simulink model "control_clean"  (R2023a)
settings: Solver=ode1be  StartTime=0.0  StopTime=tf  FixedStep=ts  RelTol=1e-3
values from neighbouring files (symbols this model uses):
  b = 0.41    [parameters.m]
  iz = 4.1    [parameters.m]
  lambda = [lambda_x; lambda_y]    [main.m]
  m = 30    [parameters.m]
  n = 501    [main.m]
  n_r_dot = -2.79    [parameters.m]
  n_v_dot = -16.41    [parameters.m]
  nrr = -3.49    [parameters.m]
  nrv = -8.8    [parameters.m]
  nvr = -8.8    [parameters.m]
  nvv = -5.49    [parameters.m]
  x = x_or    [main.m]
  x_u_dot = -2.25    [parameters.m]
  y = y_or    [main.m]
  y_r_dot = -1.31    [parameters.m]
  y_v_dot = -23.23    [parameters.m]
  yrr = -8.8    [parameters.m]
  yrv = -5.49    [parameters.m]
  yvr = -5.49    [parameters.m]
  yvv = -99.99    [parameters.m]
undefined symbols (not defined in the file or in its folder): l, m_inv
libraries: robotcorelib x1
settings Model: Creator=max  LastModifiedBy=maxpr

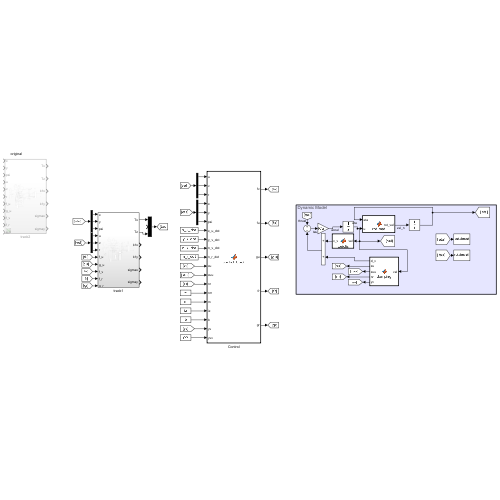
[thumbnail: Simulink's stored preview of the top-level diagram]
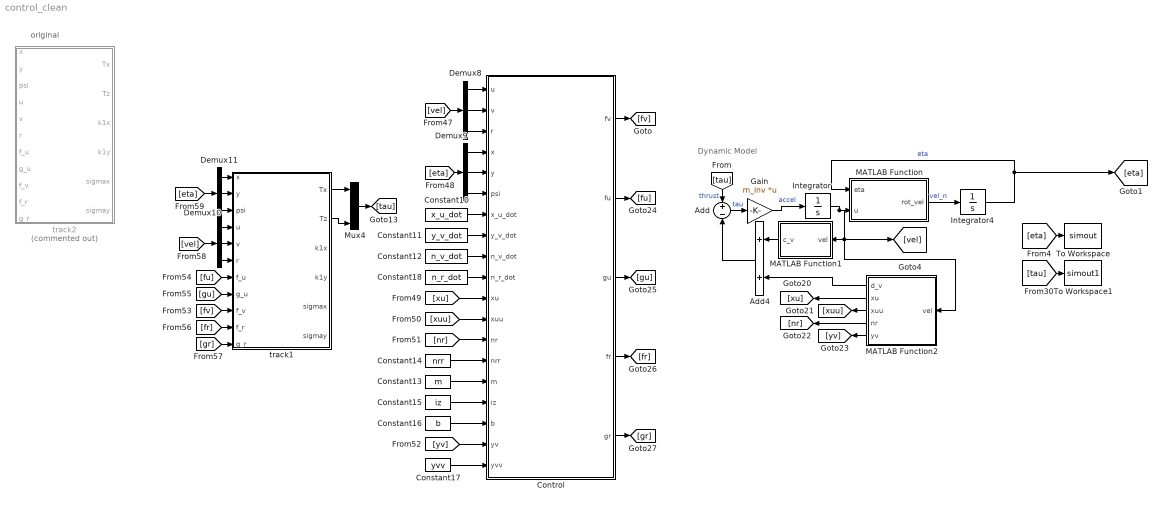
== system control_clean ==
  note: original
  note: Dynamic Model
  Add : Sum  Inputs=+|-
  Add4 : Sum
  Constant10 : Constant  Value=x_u_dot
  Constant11 : Constant  Value=y_v_dot
  Constant12 : Constant  Value=n_v_dot
  Constant13 : Constant  Value=m
  Constant14 : Constant  Value=nrr
  Constant15 : Constant  Value=iz
  Constant16 : Constant  Value=b
  Constant17 : Constant  Value=yvv
  Constant18 : Constant  Value=n_r_dot
  Control : MATLAB Function  TreatAsAtomicUnit=on
  Demux{8..11} (4 alike) : Demux  Outputs=3
  Gain : Gain  Gain=m_inv  Multiplication=Matrix(K*u)
  Integrator : Integrator  InitialCondition=[0;0;0]  UpperSaturationLimit=2.5  LowerSaturationLimit=-2.5
  Integrator4 : Integrator  InitialCondition=[0;0;0]
  MATLAB Function : MATLAB Function  TreatAsAtomicUnit=on
  MATLAB Function1 : MATLAB Function  TreatAsAtomicUnit=on
  MATLAB Function2 : MATLAB Function  TreatAsAtomicUnit=on
  Mux4 : Mux  Inputs=3
  To Workspace : ToWorkspace  VariableName=simout  SaveFormat=Timeseries  SampleTime=-1
  To Workspace1 : ToWorkspace  VariableName=simout1  SaveFormat=Timeseries  SampleTime=-1
  track1 : Subsystem
  track2 : Subsystem  Commented=on
  wires:
  Add/1 -> Gain/1  "tau"
  MATLAB Function/1(rot_vel) -> Integrator4/1  "vel_n"
  Integrator4/1 -> [eta], MATLAB Function/1(eta)  "eta"
  MATLAB Function1/1(c_v) -> Add4/1
  MATLAB Function2/1(d_v) -> Add4/2
  [eta] -> To Workspace/1
  Integrator/1 -> MATLAB Function/2(u), MATLAB Function2/1(vel), MATLAB Function1/1(vel), [vel]
  [tau] -> Add/1  "thrust"
  Gain/1 -> Integrator/1  "accel"
  [tau] -> To Workspace1/1
  Add4/1 -> Add/2
  MATLAB Function2/2(xu) -> [xu]
  MATLAB Function2/3(xuu) -> [xuu]
  MATLAB Function2/4(nr) -> [nr]
  MATLAB Function2/5(yv) -> [yv]
  [eta] -> Demux9/1
  [vel] -> Demux8/1
  Demux8/1 -> Control/1(u)
  Demux8/2 -> Control/2(v)
  Demux8/3 -> Control/3(r)
  Demux9/2 -> Control/5(y)
  Demux9/3 -> Control/6(psi)
  Demux9/1 -> Control/4(x)
  Constant10/1 -> Control/7(x_u_dot)
  Constant11/1 -> Control/8(y_v_dot)
  Constant12/1 -> Control/9(n_v_dot)
  [xu] -> Control/11(xu)
  [xuu] -> Control/12(xuu)
  [nr] -> Control/13(nr)
  Constant14/1 -> Control/14(nrr)
  Constant13/1 -> Control/15(m)
  Constant15/1 -> Control/16(iz)
  Constant16/1 -> Control/17(b)
  [yv] -> Control/18(yv)
  Constant17/1 -> Control/19(yvv)
  Control/1(fv) -> [fv]
  Control/2(fu) -> [fu]
  Control/4(fr) -> [fr]
  Control/3(gu) -> [gu]
  [fv] -> track1/9(f_v)
  [fu] -> track1/7(f_u)
  [gu] -> track1/8(g_u)
  [fr] -> track1/10(f_r)
  Constant18/1 -> Control/10(n_r_dot)
  Control/5(gr) -> [gr]
  [gr] -> track1/11(g_r)
  Demux10/1 -> track1/4(u)
  Demux10/2 -> track1/5(v)
  Demux10/3 -> track1/6(r)
  Demux11/1 -> track1/1(x)
  [eta] -> Demux11/1
  [vel] -> Demux10/1
  Demux11/2 -> track1/2(y)
  Demux11/3 -> track1/3(psi)
  Mux4/1 -> [tau]
  track1/1(Tx) -> Mux4/1
  track1/2(Tz) -> Mux4/3

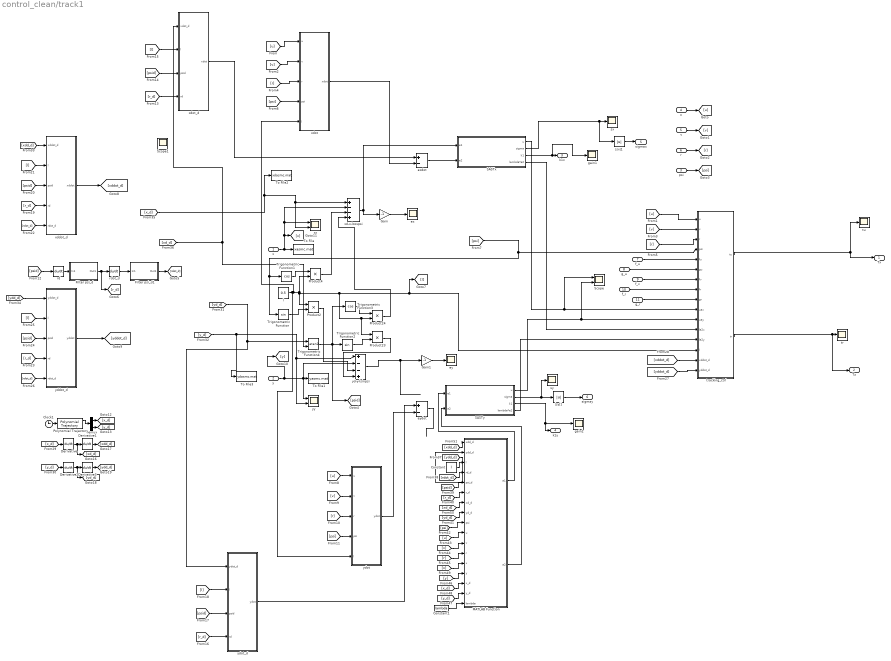
== system control_clean/track1 ==
  x : Inport
  y : Inport  Port=2
  psi : Inport  Port=3
  u : Inport  Port=4
  v : Inport  Port=5
  r : Inport  Port=6
  f_u : Inport  Port=7
  g_u : Inport  Port=8
  f_v : Inport  Port=9
  f_r : Inport  Port=10
  g_r : Inport  Port=11
  Clock1 : Clock
  Constant : Constant  Value=l
  Constant1 : Constant  Value=lambda
  Demux : Demux  Outputs=2
  Derivative{,1..3} (4 alike) : Derivative
  Filter psi_d : Subsystem
  Filter psi_d1 : Subsystem
  Gain : Gain  Gain=-1
  Gain1 : Gain  Gain=-1
  MATLAB Function : MATLAB Function  TreatAsAtomicUnit=on
  Polynomial Trajectory : robotcorelib/Polynomial Trajectory  WaypointSource=Internal  Waypoints=[x;y]  TimePoints=[t]  TimeInterval=[ 1, 4 ]  Method=Cubic Polynomial  ParameterSource=Internal  VelocityBoundaryCondition=zeros( 2, n )  AccelerationBoundaryCondition=zeros( 2, 5 )  SimulateUsing=Interpreted execution
  Product{2,4,23..24} (4 alike) : Product
  SASTx : Subsystem
  SASTy : Subsystem
  Scope : Scope  NumInputPorts=2
  Scope1 : Scope
  To File : ToFile  Filename=xasmc.mat
  To File1 : ToFile  Filename=yasmc.mat
  To File2 : ToFile  Filename=xdasmc.mat
  To File3 : ToFile  Filename=ydasmc.mat
  Trigonometric Function : Trigonometry
  Trigonometric Function1 : Trigonometry  Operator=cos
  Trigonometric Function2 : Trigonometry
  Trigonometric Function3 : Trigonometry  Operator=cos
  Trigonometric Function4 : Trigonometry  Operator=atan2
  ex : Scope
  exdot : Sum  Inputs=+-
  ey : Scope
  eydot : Sum  Inputs=+-
  gain1 : Scope
  gain2 : Scope
  l : Constant  Value=0.5
  rd : Derivative
  rdot_d : Derivative
  sx : Scope
  sy : Scope
  tr : Scope
  tracking_ctrl : MATLAB Function  TreatAsAtomicUnit=on
  tu : Scope
  xd-x-lcospsi : Sum  Inputs=+--+
  xddot_d : MATLAB Function  TreatAsAtomicUnit=on
  xdot : MATLAB Function  TreatAsAtomicUnit=on
  xdot_d : MATLAB Function  TreatAsAtomicUnit=on
  xx : Scope  NumInputPorts=2
  yd-y-lsinpsi : Sum  Inputs=+--+
  yddot_d : MATLAB Function  TreatAsAtomicUnit=on
  ydot : MATLAB Function  TreatAsAtomicUnit=on
  ydot_d : MATLAB Function  TreatAsAtomicUnit=on
  yy : Scope  NumInputPorts=2
  |sx|1 : Abs  SaturateOnIntegerOverflow=off
  |sy|1 : Abs  SaturateOnIntegerOverflow=off
  Tx : Outport
  Tz : Outport  Port=2
  k1x : Outport  Port=3  VectorParamsAs1DForOutWhenUnconnected=off
  k1y : Outport  Port=4  VectorParamsAs1DForOutWhenUnconnected=off
  sigmax : Outport  Port=5  VectorParamsAs1DForOutWhenUnconnected=off
  sigmay : Outport  Port=6  VectorParamsAs1DForOutWhenUnconnected=off
  wires:
  tracking_ctrl/2(tr) -> Tz/1, tr/1
  y/1 -> [y], yd-y-lsinpsi/2, To File1/1, yy/1
  x/1 -> [x], xd-x-lcospsi/2, xx/1, To File/1
  [x_d] -> To File2/1, xd-x-lcospsi/1, xx/2
  [y_d] -> To File3/1, yd-y-lsinpsi/1, yy/2
  xd-x-lcospsi/1 -> SASTx/1(e1), Gain/1
  [yd_d] -> ydot_d/1(ydot_d), Trigonometric Function4/1
  [xd_d] -> xdot_d/1(xdot_d), Trigonometric Function4/2
  tracking_ctrl/1(tu) -> tu/1, Tx/1
  yd-y-lsinpsi/1 -> Gain1/1
  Product2/1 -> yd-y-lsinpsi/3
  Product4/1 -> xd-x-lcospsi/3
  [psi] -> tracking_ctrl/4(psi), Trigonometric Function1/1, Trigonometric Function/1
  Trigonometric Function1/1 -> Product4/1
  Trigonometric Function/1 -> Product2/2
  SASTx/2(sigma) -> |sx|1/1, sx/1
  |sy|1/1 -> sigmay/1
  |sx|1/1 -> sigmax/1
  Trigonometric Function4/1 -> Trigonometric Function3/1, Trigonometric Function2/1, [psid]
  Trigonometric Function2/1 -> Product23/2
  Trigonometric Function3/1 -> Product24/1
  Product23/1 -> yd-y-lsinpsi/4
  Product24/1 -> xd-x-lcospsi/4
  SASTx/3(k1) -> gain1/1, k1x/1
  SASTy/2(sigma) -> sy/1, |sy|1/1
  SASTy/3(k1) -> k1y/1, gain2/1
  u/1 -> [u]
  [v] -> tracking_ctrl/2(v)
  [r] -> tracking_ctrl/3(r)
  f_u/1 -> tracking_ctrl/5(fu)
  g_u/1 -> tracking_ctrl/6(gu)
  f_v/1 -> tracking_ctrl/7(fv)
  f_r/1 -> tracking_ctrl/8(fr)
  g_r/1 -> tracking_ctrl/9(gr)
  SASTx/1(u) -> tracking_ctrl/10(uax), Scope/1
  SASTy/1(u) -> tracking_ctrl/11(uay), Scope/2
  SASTx/4(lambda*e2) -> tracking_ctrl/12(le2x)
  SASTy/4(lambda*e2) -> tracking_ctrl/13(le2y)
  eydot/1 -> ?
  exdot/1 -> SASTx/2(e2)
  xdot/1(xdot) -> exdot/2
  [u] -> xdot/1(u)
  [u] -> tracking_ctrl/1(u)
  psi/1 -> [psi]
  v/1 -> [v]
  r/1 -> [r]
  [v] -> xdot/2(v)
  [r] -> xdot/3(r)
  [psi] -> xdot/4(psi)
  ydot/1(ydot) -> eydot/2
  [r] -> ydot/3(r)
  l/1 -> ydot/5(l), xdot/5(l), [l], tracking_ctrl/14(l), Product23/1, Product24/2, Product2/1, Product4/2
  [v] -> ydot/2(v)
  [psi] -> ydot/4(psi)
  [u] -> ydot/1(u)
  xdot_d/1(xdot) -> exdot/1
  [psid] -> rd/1
  rd/1 -> Filter psi_d/1(In1)
  rdot_d/1 -> Filter psi_d1/1(In1)
  [r_d] -> xdot_d/4(rd)
  [psid] -> xdot_d/3(psid)
  [l] -> xdot_d/2(l)
  ydot_d/1(ydot) -> eydot/1
  [l] -> ydot_d/2(l)
  [r_d] -> ydot_d/4(rd)
  [psid] -> ydot_d/3(psid)
  [xdd_d] -> xddot_d/1(xddot_d)
  [l] -> xddot_d/2(l)
  [psid] -> xddot_d/3(psid)
  [r_d] -> xddot_d/4(rd)
  [rdot_d] -> xddot_d/5(rdot_d)
  xddot_d/1(xddot) -> [xddot_d]
  yddot_d/1(yddot) -> [yddot_d]
  [psid] -> yddot_d/3(psid)
  [l] -> yddot_d/2(l)
  [r_d] -> yddot_d/4(rd)
  [rdot_d] -> yddot_d/5(rdot_d)
  [ydd_d] -> yddot_d/1(yddot_d)
  [yddot_d] -> tracking_ctrl/16(yddot_d)
  [xddot_d] -> tracking_ctrl/15(xddot_d)
  Filter psi_d/1(Out1) -> [r_d], rdot_d/1
  Filter psi_d1/1(Out1) -> [rdot_d]
  Gain/1 -> ex/1
  Gain1/1 -> ey/1
  Demux/1 -> [x_d]
  Polynomial Trajectory/1 -> Demux/1
  Clock1/1 -> Polynomial Trajectory/1
  Demux/2 -> [y_d]
  [x_d] -> Derivative/1
  Derivative/1 -> [xd_d], Derivative1/1
  Derivative1/1 -> [xdd_d]
  [y_d] -> Derivative2/1
  Derivative3/1 -> [ydd_d]
  Derivative2/1 -> [yd_d], Derivative3/1
  Constant/1 -> MATLAB Function/3(l)
  [ydd_d] -> MATLAB Function/2(ydd_d)
  [rdot_d] -> MATLAB Function/4(rd_d)
  [psid] -> MATLAB Function/5(psi_d)
  [r_d] -> MATLAB Function/6(r_d)
  [yd_d] -> MATLAB Function/8(yd_d)
  [psi] -> MATLAB Function/9(psi)
  [u] -> MATLAB Function/10(u)
  [v] -> MATLAB Function/11(v)
  [r] -> MATLAB Function/12(r)
  [y] -> MATLAB Function/14(y)
  MATLAB Function/1(e1) -> SASTy/1(e1)
  MATLAB Function/2(e2) -> SASTy/2(e2)
  [y_d] -> MATLAB Function/16(y_d)
  [x_d] -> MATLAB Function/15(x_d)
  [x] -> MATLAB Function/13(x)
  [xd_d] -> MATLAB Function/7(xd_d)
  [xdd_d] -> MATLAB Function/1(xdd_d)
  Constant1/1 -> MATLAB Function/17(lambda)

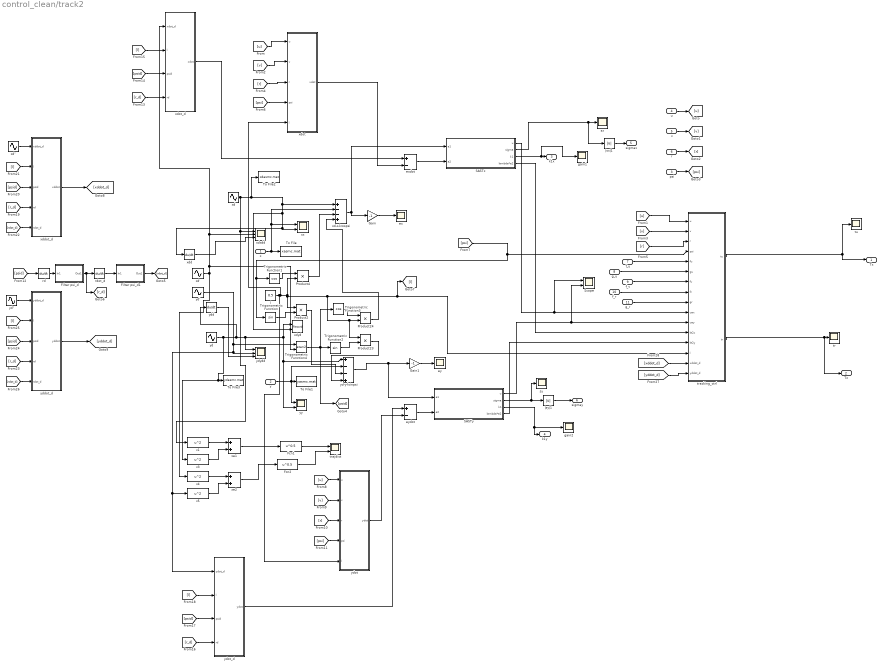
== system control_clean/track2 ==
  x : Inport
  y : Inport  Port=2
  psi : Inport  Port=3
  u : Inport  Port=4
  v : Inport  Port=5
  r : Inport  Port=6
  f_u : Inport  Port=7
  g_u : Inport  Port=8
  f_v : Inport  Port=9
  f_r : Inport  Port=10
  g_r : Inport  Port=11
  Fcn1 : Fcn  Expr=u^0.5
  Fcn2 : Fcn  Expr=u^0.5
  Filter psi_d : Subsystem
  Filter psi_d1 : Subsystem
  Gain : Gain  Gain=-1
  Gain1 : Gain  Gain=-1
  Product{2,4,23..24} (4 alike) : Product
  SASTx : Subsystem
  SASTy : Subsystem
  Scope : Scope  NumInputPorts=2
  To File : ToFile  Filename=xasmc.mat
  To File1 : ToFile  Filename=yasmc.mat
  To File2 : ToFile  Filename=xdasmc.mat
  To File3 : ToFile  Filename=ydasmc.mat
  Trigonometric Function : Trigonometry
  Trigonometric Function1 : Trigonometry  Operator=cos
  Trigonometric Function2 : Trigonometry
  Trigonometric Function3 : Trigonometry  Operator=cos
  Trigonometric Function4 : Trigonometry  Operator=atan2
  ex : Scope
  exdot : Sum  Inputs=+-
  ey : Scope
  eydot : Sum  Inputs=+-
  gain1 : Scope
  gain2 : Scope
  l : Constant  Value=0.5
  rd : Derivative
  rdot_d : Derivative
  sx : Scope
  sy : Scope
  tr : Scope
  tracking_ctrl : MATLAB Function  TreatAsAtomicUnit=on
  trajdist : Scope  NumInputPorts=2
  tu : Scope
  v{1,3..5} (4 alike) : Fcn  Expr=u^2
  xd : Sin  Amplitude=2.5  Bias=0.5  Frequency=pi/15  SampleTime=0
  xd' : Sin  Amplitude=2.5*pi/15  Frequency=pi/15  Phase=pi/2  SampleTime=0
  xd'' : Sin  Amplitude=-2.5*(pi/15)*(pi/15)  Frequency=pi/15  SampleTime=0
  xd-x-lcospsi : Sum  Inputs=+--+
  xdd : Derivative
  xddot_d : MATLAB Function  TreatAsAtomicUnit=on
  xdot : MATLAB Function  TreatAsAtomicUnit=on
  xdot_d : MATLAB Function  TreatAsAtomicUnit=on
  xdxdd : Scope  NumInputPorts=3
  xdyd : Record  FileSettingsInternal="{\"entries\":[{\"content\":{\"excelSettings\":{\"content\":{},\"type\":\"Streamout.ExcelSettings\"}},\"type\":\"Streamout.FileSettingStorage\",\"uuid\":\"\"}],\"packageUris\":[\"http:\\/\\/schema.mathworks.com\\/mf0\\/streamout_blocks\\/R2020a\"],\"version\":\"1.0\"}"  Layout=[1 1]  SignalsInternal="{\"entries\":[{\"content\":{\"signals\":[{\"content\":{\"blockPath\":[],\"dimensions\":[1],\"domain\":\"\",\"lineColor\":\"#a2142f\",\"plots\":[1],\"port\":1,\"signalID\":8,\"signalName\":\"yd\"},\"type\":\"RecordBlkView.Signal\",\"uuid\":\"\"},{\"content\":{\"blockPath\":[],\"dimensions\":[1],\"domain\":\"\",\"lineColor\":\"#139fff\",\"plots\":[1],\"port\":2,\"signalID\":11,\"signalName\":\"xd\"},\"type\":\"RecordBlkView.Signal\",\"uuid\":\"\"}]},\"type\":\"RecordBlkView.InputSignals\",\"uuid\":\"\"}],\"packageUris\":[\"http:\\/\\/schema.mathworks.com\\/mf0\\/streamout_blocks\\/R2020a\"],\"version\":\"1.0\"}"  VisualizationBindings="{\"xyplotplugin\":{\"info\":[{\"series\":[{\"bindingParametersList\":[{\"parameter\":\"X-Axis\",\"signalID\":8,\"signalName\":\"yd\"},{\"parameter\":\"Y-Axis\",\"signalID\":11,\"signalName\":\"xd\"}],\"seriesID\":30671}],\"subplotID\":1}]}}"  CompatibilityTag=XY  st=-1
  xe1 : Sum
  xe2 : Sum
  xx : Scope  NumInputPorts=2
  yd : Sin  Amplitude=7  Bias=-7.5  Frequency=pi/30  Phase=pi/2  SampleTime=0
  yd' : Sin  Amplitude=-7*pi/30  Frequency=pi/30  SampleTime=0
  yd'' : Sin  Amplitude=-7*(pi/30)*(pi/30)  Frequency=pi/30  Phase=pi/2  SampleTime=0
  yd-y-lsinpsi : Sum  Inputs=+--+
  ydd : Derivative
  yddot_d : MATLAB Function  TreatAsAtomicUnit=on
  ydot : MATLAB Function  TreatAsAtomicUnit=on
  ydot_d : MATLAB Function  TreatAsAtomicUnit=on
  ydydd : Scope  NumInputPorts=3
  yy : Scope  NumInputPorts=2
  |sx|1 : Abs  SaturateOnIntegerOverflow=off
  |sy|1 : Abs  SaturateOnIntegerOverflow=off
  Tx : Outport
  Tz : Outport  Port=2
  k1x : Outport  Port=3  VectorParamsAs1DForOutWhenUnconnected=off
  k1y : Outport  Port=4  VectorParamsAs1DForOutWhenUnconnected=off
  sigmax : Outport  Port=5  VectorParamsAs1DForOutWhenUnconnected=off
  sigmay : Outport  Port=6  VectorParamsAs1DForOutWhenUnconnected=off
  wires:
  Gain1/1 -> ey/1
  Gain/1 -> ex/1
  Filter psi_d1/1(Out1) -> [rdot_d]
  Filter psi_d/1(Out1) -> rdot_d/1, [r_d]
  [xddot_d] -> tracking_ctrl/15(xddot_d)
  [yddot_d] -> tracking_ctrl/16(yddot_d)
  yd''/1 -> yddot_d/1(yddot_d)
  [rdot_d] -> yddot_d/5(rdot_d)
  [r_d] -> yddot_d/4(rd)
  [l] -> yddot_d/2(l)
  [psid] -> yddot_d/3(psid)
  yddot_d/1(yddot) -> [yddot_d]
  xddot_d/1(xddot) -> [xddot_d]
  [rdot_d] -> xddot_d/5(rdot_d)
  [r_d] -> xddot_d/4(rd)
  [psid] -> xddot_d/3(psid)
  [l] -> xddot_d/2(l)
  xd''/1 -> xddot_d/1(xddot_d)
  [psid] -> ydot_d/3(psid)
  [r_d] -> ydot_d/4(rd)
  [l] -> ydot_d/2(l)
  ydot_d/1(ydot) -> eydot/1
  [l] -> xdot_d/2(l)
  [psid] -> xdot_d/3(psid)
  [r_d] -> xdot_d/4(rd)
  rdot_d/1 -> Filter psi_d1/1(In1)
  rd/1 -> Filter psi_d/1(In1)
  [psid] -> rd/1
  xdot_d/1(xdot) -> exdot/1
  [u] -> ydot/1(u)
  [psi] -> ydot/4(psi)
  [v] -> ydot/2(v)
  l/1 -> Product4/2, Product2/1, Product24/2, Product23/1, tracking_ctrl/14(l), [l], xdot/5(l), ydot/5(l)
  [r] -> ydot/3(r)
  ydot/1(ydot) -> eydot/2
  [psi] -> xdot/4(psi)
  [r] -> xdot/3(r)
  [v] -> xdot/2(v)
  r/1 -> [r]
  v/1 -> [v]
  psi/1 -> [psi]
  [u] -> tracking_ctrl/1(u)
  [u] -> xdot/1(u)
  xdot/1(xdot) -> exdot/2
  exdot/1 -> SASTx/2(e2)
  eydot/1 -> SASTy/2(e2)
  SASTy/4(lambda*e2) -> tracking_ctrl/13(le2y)
  SASTx/4(lambda*e2) -> tracking_ctrl/12(le2x)
  SASTy/1(u) -> Scope/2, tracking_ctrl/11(uay)
  SASTx/1(u) -> Scope/1, tracking_ctrl/10(uax)
  g_r/1 -> tracking_ctrl/9(gr)
  f_r/1 -> tracking_ctrl/8(fr)
  f_v/1 -> tracking_ctrl/7(fv)
  g_u/1 -> tracking_ctrl/6(gu)
  f_u/1 -> tracking_ctrl/5(fu)
  [r] -> tracking_ctrl/3(r)
  [v] -> tracking_ctrl/2(v)
  u/1 -> [u]
  SASTy/3(k1) -> gain2/1, k1y/1
  SASTy/2(sigma) -> |sy|1/1, sy/1
  SASTx/3(k1) -> k1x/1, gain1/1
  Product24/1 -> xd-x-lcospsi/4
  Product23/1 -> yd-y-lsinpsi/4
  Trigonometric Function3/1 -> Product24/1
  Trigonometric Function2/1 -> Product23/2
  Trigonometric Function4/1 -> [psid], Trigonometric Function2/1, Trigonometric Function3/1
  |sx|1/1 -> sigmax/1
  |sy|1/1 -> sigmay/1
  SASTx/2(sigma) -> sx/1, |sx|1/1
  Trigonometric Function/1 -> Product2/2
  Trigonometric Function1/1 -> Product4/1
  [psi] -> Trigonometric Function/1, Trigonometric Function1/1, tracking_ctrl/4(psi)
  Product4/1 -> xd-x-lcospsi/3
  Product2/1 -> yd-y-lsinpsi/3
  yd-y-lsinpsi/1 -> Gain1/1, SASTy/1(e1)
  v5/1 -> xe2/2
  v4/1 -> xe2/1
  xe2/1 -> Fcn2/1
  v3/1 -> xe1/2
  v1/1 -> xe1/1
  xe1/1 -> Fcn1/1
  Fcn2/1 -> trajdist/2
  Fcn1/1 -> trajdist/1
  xdd/1 -> xdxdd/3
  ydd/1 -> ydydd/3
  tracking_ctrl/1(tu) -> Tx/1, tu/1
  xd'/1 -> v4/1, Trigonometric Function4/2, xdxdd/2, xdot_d/1(xdot_d)
  yd'/1 -> Trigonometric Function4/1, v5/1, ydot_d/1(ydot_d), ydydd/2
  xd-x-lcospsi/1 -> Gain/1, SASTx/1(e1)
  yd/1 -> ydd/1, ydydd/1, xdyd/1, yy/2, yd-y-lsinpsi/1, To File3/1, v3/1
  xd/1 -> xdyd/2, xdd/1, xx/2, xd-x-lcospsi/1, To File2/1, xdxdd/1, v1/1
  x/1 -> To File/1, xx/1, xd-x-lcospsi/2
  y/1 -> yy/1, To File1/1, yd-y-lsinpsi/2
  tracking_ctrl/2(tr) -> tr/1, Tz/1

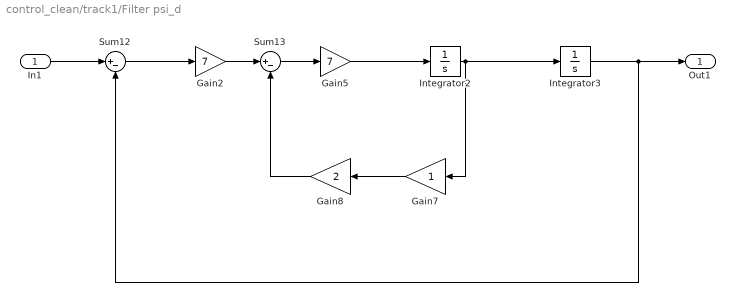
== system control_clean/track1/Filter psi_d ==
  In1 : Inport
  Gain2 : Gain  Gain=7
  Gain5 : Gain  Gain=7
  Gain7 : Gain
  Gain8 : Gain  Gain=2
  Integrator2 : Integrator
  Integrator3 : Integrator
  Sum12 : Sum  Inputs=|+-
  Sum13 : Sum  Inputs=|+-
  Out1 : Outport  VectorParamsAs1DForOutWhenUnconnected=off
  wires:
  Gain7/1 -> Gain8/1
  Sum12/1 -> Gain2/1
  Integrator3/1 -> Out1/1, Sum12/2
  In1/1 -> Sum12/1
  Gain2/1 -> Sum13/1
  Gain5/1 -> Integrator2/1
  Sum13/1 -> Gain5/1
  Gain8/1 -> Sum13/2
  Integrator2/1 -> Gain7/1, Integrator3/1

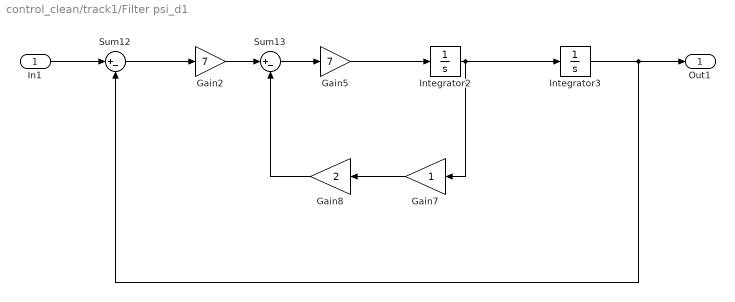
== system control_clean/track1/Filter psi_d1 ==
  In1 : Inport
  Gain2 : Gain  Gain=7
  Gain5 : Gain  Gain=7
  Gain7 : Gain
  Gain8 : Gain  Gain=2
  Integrator2 : Integrator
  Integrator3 : Integrator
  Sum12 : Sum  Inputs=|+-
  Sum13 : Sum  Inputs=|+-
  Out1 : Outport  VectorParamsAs1DForOutWhenUnconnected=off
  wires:
  Gain7/1 -> Gain8/1
  Sum12/1 -> Gain2/1
  Integrator3/1 -> Out1/1, Sum12/2
  In1/1 -> Sum12/1
  Gain2/1 -> Sum13/1
  Gain5/1 -> Integrator2/1
  Sum13/1 -> Gain5/1
  Gain8/1 -> Sum13/2
  Integrator2/1 -> Gain7/1, Integrator3/1

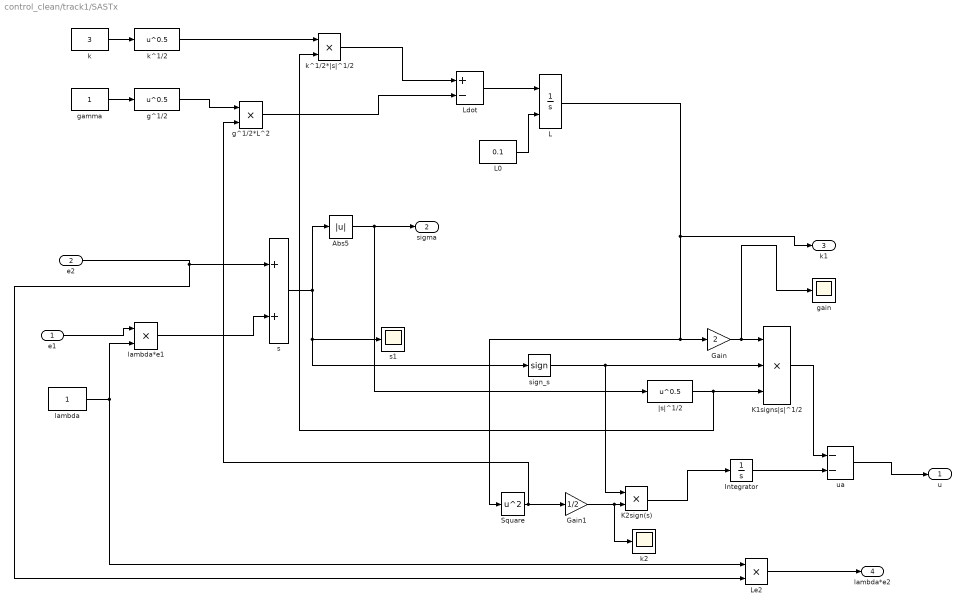
== system control_clean/track1/SASTx ==
  e1 : Inport
  e2 : Inport  Port=2
  Abs5 : Abs  SaturateOnIntegerOverflow=off
  Gain : Gain  Gain=2
  Gain1 : Gain  Gain=1/2
  Integrator : Integrator
  K1signs|s|^1/2 : Product  Inputs=***
  K2sign(s) : Product
  L : Integrator  InitialConditionSource=external
  L0 : Constant  Value=0.1
  Ldot : Sum  Inputs=+-
  Le2 : Product
  Square : Math  Operator=square
  g^1/2 : Fcn  Expr=u^0.5
  g^1/2*L^2 : Product
  gain : Scope
  gamma : Constant
  k : Constant  Value=3
  k2 : Scope
  k^1/2 : Fcn  Expr=u^0.5
  k^1/2*|s|^1/2 : Product
  lambda : Constant
  lambda*e1 : Product
  s : Sum
  s1 : Scope
  sign_s : Signum
  ua : Sum  Inputs=--
  |s|^1/2 : Fcn  Expr=u^0.5
  u : Outport  VectorParamsAs1DForOutWhenUnconnected=off
  sigma : Outport  Port=2  VectorParamsAs1DForOutWhenUnconnected=off
  k1 : Outport  Port=3  VectorParamsAs1DForOutWhenUnconnected=off
  lambda*e2 : Outport  Port=4  VectorParamsAs1DForOutWhenUnconnected=off
  wires:
  s/1 -> s1/1, sign_s/1, Abs5/1
  sign_s/1 -> K2sign(s)/1, K1signs|s|^1/2/2
  K1signs|s|^1/2/1 -> ua/1
  Abs5/1 -> |s|^1/2/1, sigma/1
  |s|^1/2/1 -> k^1/2*|s|^1/2/2, K1signs|s|^1/2/3
  Le2/1 -> lambda*e2/1
  e2/1 -> Le2/2, s/1
  lambda/1 -> Le2/1, lambda*e1/2
  e1/1 -> lambda*e1/1
  lambda*e1/1 -> s/2
  L/1 -> k1/1, Gain/1, Square/1
  ua/1 -> u/1
  Gain/1 -> gain/1, K1signs|s|^1/2/1
  Integrator/1 -> ua/2
  K2sign(s)/1 -> Integrator/1
  Square/1 -> g^1/2*L^2/2, Gain1/1
  Gain1/1 -> k2/1, K2sign(s)/2
  Ldot/1 -> L/1
  L0/1 -> L/2
  k/1 -> k^1/2/1
  gamma/1 -> g^1/2/1
  g^1/2/1 -> g^1/2*L^2/1
  k^1/2/1 -> k^1/2*|s|^1/2/1
  g^1/2*L^2/1 -> Ldot/2
  k^1/2*|s|^1/2/1 -> Ldot/1

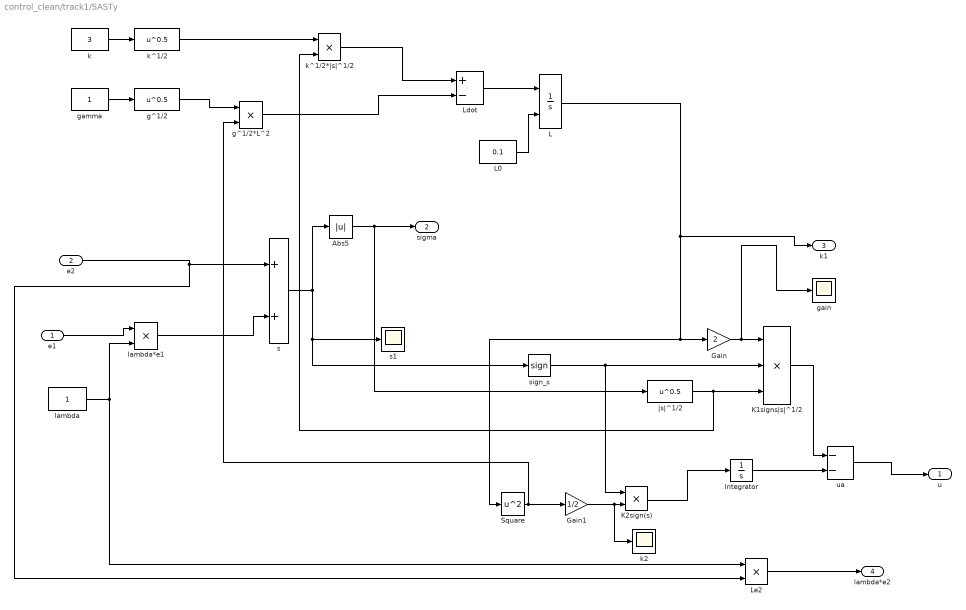
== system control_clean/track1/SASTy ==
  e1 : Inport
  e2 : Inport  Port=2
  Abs5 : Abs  SaturateOnIntegerOverflow=off
  Gain : Gain  Gain=2
  Gain1 : Gain  Gain=1/2
  Integrator : Integrator
  K1signs|s|^1/2 : Product  Inputs=***
  K2sign(s) : Product
  L : Integrator  InitialConditionSource=external
  L0 : Constant  Value=0.1
  Ldot : Sum  Inputs=+-
  Le2 : Product
  Square : Math  Operator=square
  g^1/2 : Fcn  Expr=u^0.5
  g^1/2*L^2 : Product
  gain : Scope
  gamma : Constant
  k : Constant  Value=3
  k2 : Scope
  k^1/2 : Fcn  Expr=u^0.5
  k^1/2*|s|^1/2 : Product
  lambda : Constant
  lambda*e1 : Product
  s : Sum
  s1 : Scope
  sign_s : Signum
  ua : Sum  Inputs=--
  |s|^1/2 : Fcn  Expr=u^0.5
  u : Outport  VectorParamsAs1DForOutWhenUnconnected=off
  sigma : Outport  Port=2  VectorParamsAs1DForOutWhenUnconnected=off
  k1 : Outport  Port=3  VectorParamsAs1DForOutWhenUnconnected=off
  lambda*e2 : Outport  Port=4  VectorParamsAs1DForOutWhenUnconnected=off
  wires:
  s/1 -> s1/1, sign_s/1, Abs5/1
  sign_s/1 -> K2sign(s)/1, K1signs|s|^1/2/2
  K1signs|s|^1/2/1 -> ua/1
  Abs5/1 -> |s|^1/2/1, sigma/1
  |s|^1/2/1 -> k^1/2*|s|^1/2/2, K1signs|s|^1/2/3
  Le2/1 -> lambda*e2/1
  e2/1 -> Le2/2, s/1
  lambda/1 -> Le2/1, lambda*e1/2
  e1/1 -> lambda*e1/1
  lambda*e1/1 -> s/2
  L/1 -> k1/1, Gain/1, Square/1
  ua/1 -> u/1
  Gain/1 -> gain/1, K1signs|s|^1/2/1
  Integrator/1 -> ua/2
  K2sign(s)/1 -> Integrator/1
  Square/1 -> g^1/2*L^2/2, Gain1/1
  Gain1/1 -> k2/1, K2sign(s)/2
  Ldot/1 -> L/1
  L0/1 -> L/2
  k/1 -> k^1/2/1
  gamma/1 -> g^1/2/1
  g^1/2/1 -> g^1/2*L^2/1
  k^1/2/1 -> k^1/2*|s|^1/2/1
  g^1/2*L^2/1 -> Ldot/2
  k^1/2*|s|^1/2/1 -> Ldot/1

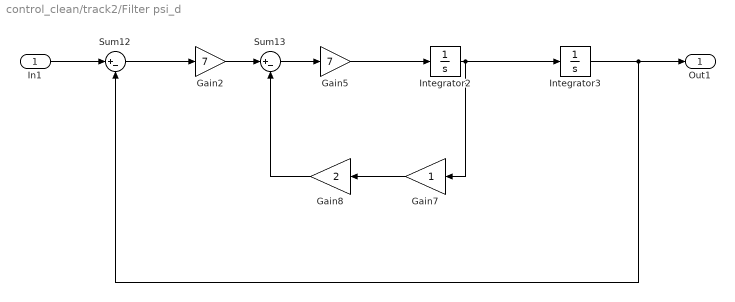
== system control_clean/track2/Filter psi_d ==
  In1 : Inport
  Gain2 : Gain  Gain=7
  Gain5 : Gain  Gain=7
  Gain7 : Gain
  Gain8 : Gain  Gain=2
  Integrator2 : Integrator
  Integrator3 : Integrator
  Sum12 : Sum  Inputs=|+-
  Sum13 : Sum  Inputs=|+-
  Out1 : Outport  VectorParamsAs1DForOutWhenUnconnected=off
  wires:
  Integrator2/1 -> Integrator3/1, Gain7/1
  Gain8/1 -> Sum13/2
  Sum13/1 -> Gain5/1
  Gain5/1 -> Integrator2/1
  Gain2/1 -> Sum13/1
  In1/1 -> Sum12/1
  Integrator3/1 -> Sum12/2, Out1/1
  Sum12/1 -> Gain2/1
  Gain7/1 -> Gain8/1

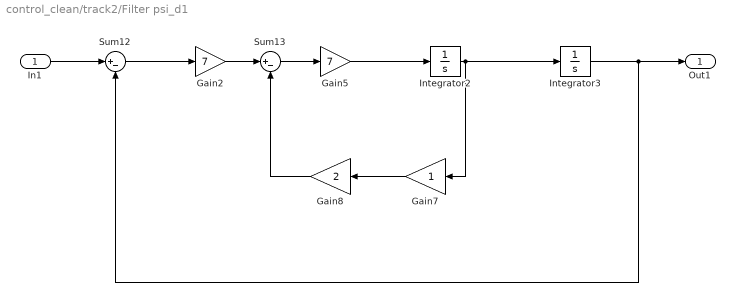
== system control_clean/track2/Filter psi_d1 ==
  In1 : Inport
  Gain2 : Gain  Gain=7
  Gain5 : Gain  Gain=7
  Gain7 : Gain
  Gain8 : Gain  Gain=2
  Integrator2 : Integrator
  Integrator3 : Integrator
  Sum12 : Sum  Inputs=|+-
  Sum13 : Sum  Inputs=|+-
  Out1 : Outport  VectorParamsAs1DForOutWhenUnconnected=off
  wires:
  Integrator2/1 -> Integrator3/1, Gain7/1
  Gain8/1 -> Sum13/2
  Sum13/1 -> Gain5/1
  Gain5/1 -> Integrator2/1
  Gain2/1 -> Sum13/1
  In1/1 -> Sum12/1
  Integrator3/1 -> Sum12/2, Out1/1
  Sum12/1 -> Gain2/1
  Gain7/1 -> Gain8/1

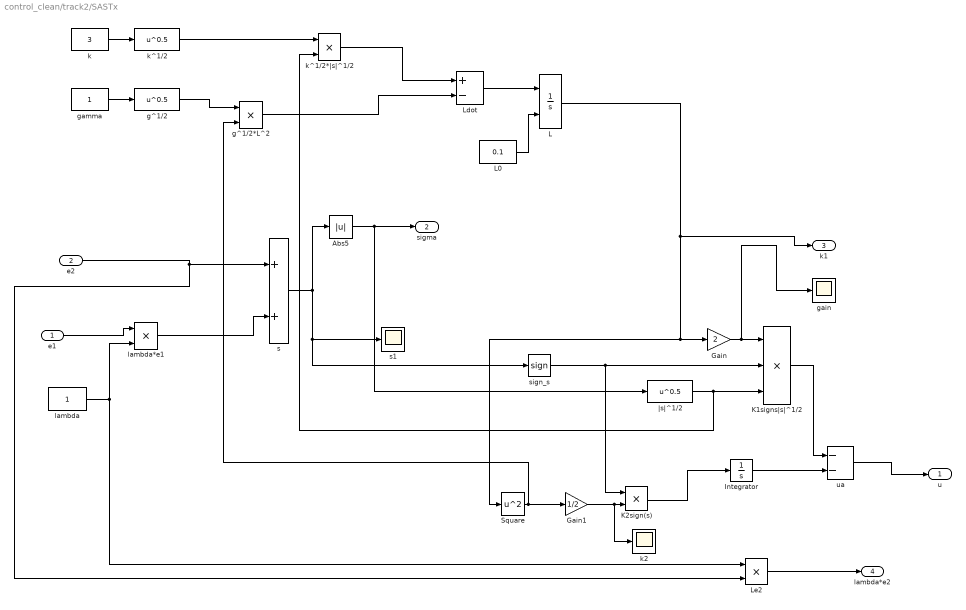
== system control_clean/track2/SASTx ==
  e1 : Inport
  e2 : Inport  Port=2
  Abs5 : Abs  SaturateOnIntegerOverflow=off
  Gain : Gain  Gain=2
  Gain1 : Gain  Gain=1/2
  Integrator : Integrator
  K1signs|s|^1/2 : Product  Inputs=***
  K2sign(s) : Product
  L : Integrator  InitialConditionSource=external
  L0 : Constant  Value=0.1
  Ldot : Sum  Inputs=+-
  Le2 : Product
  Square : Math  Operator=square
  g^1/2 : Fcn  Expr=u^0.5
  g^1/2*L^2 : Product
  gain : Scope
  gamma : Constant
  k : Constant  Value=3
  k2 : Scope
  k^1/2 : Fcn  Expr=u^0.5
  k^1/2*|s|^1/2 : Product
  lambda : Constant
  lambda*e1 : Product
  s : Sum
  s1 : Scope
  sign_s : Signum
  ua : Sum  Inputs=--
  |s|^1/2 : Fcn  Expr=u^0.5
  u : Outport  VectorParamsAs1DForOutWhenUnconnected=off
  sigma : Outport  Port=2  VectorParamsAs1DForOutWhenUnconnected=off
  k1 : Outport  Port=3  VectorParamsAs1DForOutWhenUnconnected=off
  lambda*e2 : Outport  Port=4  VectorParamsAs1DForOutWhenUnconnected=off
  wires:
  k^1/2*|s|^1/2/1 -> Ldot/1
  g^1/2*L^2/1 -> Ldot/2
  k^1/2/1 -> k^1/2*|s|^1/2/1
  g^1/2/1 -> g^1/2*L^2/1
  gamma/1 -> g^1/2/1
  k/1 -> k^1/2/1
  L0/1 -> L/2
  Ldot/1 -> L/1
  Gain1/1 -> K2sign(s)/2, k2/1
  Square/1 -> Gain1/1, g^1/2*L^2/2
  K2sign(s)/1 -> Integrator/1
  Integrator/1 -> ua/2
  Gain/1 -> K1signs|s|^1/2/1, gain/1
  ua/1 -> u/1
  L/1 -> Square/1, Gain/1, k1/1
  lambda*e1/1 -> s/2
  e1/1 -> lambda*e1/1
  lambda/1 -> lambda*e1/2, Le2/1
  e2/1 -> s/1, Le2/2
  Le2/1 -> lambda*e2/1
  |s|^1/2/1 -> K1signs|s|^1/2/3, k^1/2*|s|^1/2/2
  Abs5/1 -> sigma/1, |s|^1/2/1
  K1signs|s|^1/2/1 -> ua/1
  sign_s/1 -> K1signs|s|^1/2/2, K2sign(s)/1
  s/1 -> Abs5/1, sign_s/1, s1/1

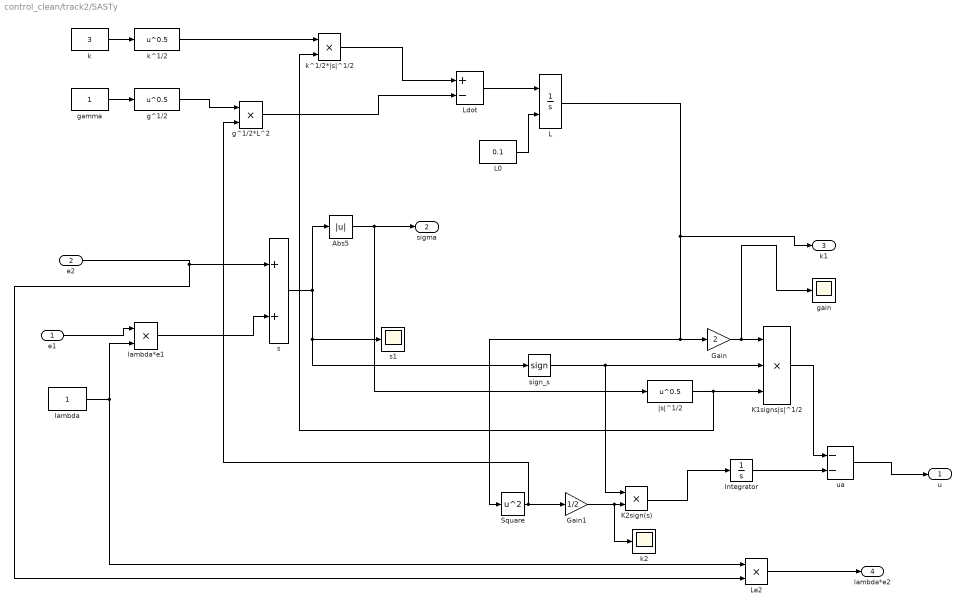
== system control_clean/track2/SASTy ==
  e1 : Inport
  e2 : Inport  Port=2
  Abs5 : Abs  SaturateOnIntegerOverflow=off
  Gain : Gain  Gain=2
  Gain1 : Gain  Gain=1/2
  Integrator : Integrator
  K1signs|s|^1/2 : Product  Inputs=***
  K2sign(s) : Product
  L : Integrator  InitialConditionSource=external
  L0 : Constant  Value=0.1
  Ldot : Sum  Inputs=+-
  Le2 : Product
  Square : Math  Operator=square
  g^1/2 : Fcn  Expr=u^0.5
  g^1/2*L^2 : Product
  gain : Scope
  gamma : Constant
  k : Constant  Value=3
  k2 : Scope
  k^1/2 : Fcn  Expr=u^0.5
  k^1/2*|s|^1/2 : Product
  lambda : Constant
  lambda*e1 : Product
  s : Sum
  s1 : Scope
  sign_s : Signum
  ua : Sum  Inputs=--
  |s|^1/2 : Fcn  Expr=u^0.5
  u : Outport  VectorParamsAs1DForOutWhenUnconnected=off
  sigma : Outport  Port=2  VectorParamsAs1DForOutWhenUnconnected=off
  k1 : Outport  Port=3  VectorParamsAs1DForOutWhenUnconnected=off
  lambda*e2 : Outport  Port=4  VectorParamsAs1DForOutWhenUnconnected=off
  wires:
  k^1/2*|s|^1/2/1 -> Ldot/1
  g^1/2*L^2/1 -> Ldot/2
  k^1/2/1 -> k^1/2*|s|^1/2/1
  g^1/2/1 -> g^1/2*L^2/1
  gamma/1 -> g^1/2/1
  k/1 -> k^1/2/1
  L0/1 -> L/2
  Ldot/1 -> L/1
  Gain1/1 -> K2sign(s)/2, k2/1
  Square/1 -> Gain1/1, g^1/2*L^2/2
  K2sign(s)/1 -> Integrator/1
  Integrator/1 -> ua/2
  Gain/1 -> K1signs|s|^1/2/1, gain/1
  ua/1 -> u/1
  L/1 -> Square/1, Gain/1, k1/1
  lambda*e1/1 -> s/2
  e1/1 -> lambda*e1/1
  lambda/1 -> lambda*e1/2, Le2/1
  e2/1 -> s/1, Le2/2
  Le2/1 -> lambda*e2/1
  |s|^1/2/1 -> K1signs|s|^1/2/3, k^1/2*|s|^1/2/2
  Abs5/1 -> sigma/1, |s|^1/2/1
  K1signs|s|^1/2/1 -> ua/1
  sign_s/1 -> K1signs|s|^1/2/2, K2sign(s)/1
  s/1 -> Abs5/1, sign_s/1, s1/1

== matlab function control_clean/track2/xdot ==
  data: u input; v input; r input; psi input; xdot output; l input
function xdot   = fcn(u, v, r, psi, l)
xdot = u*cos(psi)-v*sin(psi)-r*l*sin(psi);

== matlab function control_clean/track2/xdot_d ==
  data: xdot_d input; l input; psid input; rd input; xdot output
function xdot   = fcn(xdot_d, l, psid, rd)
xdot = xdot_d - l*sin(psid)*rd;

== matlab function control_clean/track2/yddot_d ==
  data: yddot_d input; l input; psid input; rd input; yddot output; rdot_d input
function yddot   = fcn(yddot_d, l, psid, rd, rdot_d)
yddot = yddot_d + l*cos(psid)*rdot_d - l*sin(psid)*rd*rd;

== matlab function control_clean/track2/ydot ==
  data: u input; v input; r input; psi input; ydot output; l input
function ydot   = fcn(u, v, r, psi, l)
ydot = u*sin(psi)+v*cos(psi)+r*l*cos(psi);

== matlab function control_clean/track2/ydot_d ==
  data: ydot_d input; l input; psid input; rd input; ydot output
function ydot   = fcn(ydot_d, l, psid, rd)
ydot = ydot_d + l*cos(psid)*rd;

== matlab function control_clean/track1/MATLAB Function ==
  data: xdd_d input; ydd_d input; e1 output; l input; rd_d input; psi_d input; r_d input; xd_d input; yd_d input; psi input; u input; v input; r input; x input; y input; x_d input; e2 output; y_d input; lambda input
function [e1,e2]= fcn(xdd_d, ydd_d, l, rd_d, psi_d, r_d, xd_d, yd_d, psi, u, v, r, x, y, x_d, y_d, lambda)
xddot_d = xdd_d - l*sin(psi_d)*rd_d - l*cos(psi_d)*r_d^2;
yddot_d = ydd_d + l*cos(rd_d) - l*sin(psi_d)*r_d^2;

xd_d = xd_d - l*sin(psi_d)*r_d;
xd = u*cos(psi) - v*sin(psi) - r*l*sin(psi);
yd_d = yd_d + l*cos(psi_d)*r_d;
yd = u*sin(psi) + v*cos(psi) + r*l*cos(psi);

e1x = x_d + l*cos(psi_d) - (x + l*cos(psi));
e2x = xd_d - xd;
e1y = y_d + l*sin(psi_d) - (y + l*sin(psi));
e2y = yd_d - yd;
e1 = [e1x; e1y];
e2 = [e2x; e2y];

s = lambda.*e1 + e2;

== matlab function control_clean/Control ==
  data: u input; fv output; v input; r input; x input; y input; psi input; x_u_dot input; y_v_dot input; n_v_dot input; n_r_dot input; xu input; xuu input; nr input; nrr input; m input; iz input; b input; yv input; yvv input; fu output; gu output; fr output; gr output
function [fv,fu,gu,fr, gr]= control_block(u,v,r,x,y,psi,x_u_dot,y_v_dot,n_v_dot, n_r_dot,xu,xuu,nr,nrr,m,iz,b,yv,yvv)
fv = ((-m+x_u_dot)*u*r + (yvv*v*abs(v)+yv*abs(v)))/(m-y_v_dot);
fu = ((m-y_v_dot)*v*r + (xuu*u*abs(u) + xu*abs(u)))/(m-x_u_dot);
gu = 1/(m-x_u_dot);
fr = ((-x_u_dot + y_v_dot)*u*v + nr*r + nrr*r*abs(r))/(iz - n_r_dot);
gr = 1/(iz - n_r_dot);

== matlab function control_clean/track1/tracking_ctrl ==
  data: u input; v input; r input; psi input; tu output; fu input; gu input; fv input; fr input; gr input; uax input; uay input; le2x input; le2y input; tr output; l input; xddot_d input; yddot_d input
function [tu,tr]  = fcn(u, v, r, psi, fu, gu, fv, fr, gr, uax, uay, le2x, le2y, l, xddot_d, yddot_d)
gz = [gu*cos(psi), -gr*l*sin(psi); gu*sin(psi), gr*l*cos(psi)];
lep = [le2x; le2y];
f1 = [cos(psi), -sin(psi); sin(psi), cos(psi)];
f2 = [fu - v*r - l*r*r; u*r + fv + l*fr];
fz = f1*f2;
ua = [uax; uay];
ref_ddot = [xddot_d; yddot_d];
uz = inv(gz)*(ref_ddot + lep - fz - ua);
tu = uz(1);
tr = uz(2);

== matlab function control_clean/track1/xddot_d ==
  data: xddot_d input; l input; psid input; rd input; xddot output; rdot_d input
function xddot   = fcn(xddot_d, l, psid, rd, rdot_d)
xddot = xddot_d - l*sin(psid)*rdot_d - l*cos(psid)*rd*rd;

== matlab function control_clean/track1/xdot ==
  data: u input; v input; r input; psi input; xdot output; l input
function xdot   = fcn(u, v, r, psi, l)
xdot = u*cos(psi)-v*sin(psi)-r*l*sin(psi);

== matlab function control_clean/track1/xdot_d ==
  data: xdot_d input; l input; psid input; rd input; xdot output
function xdot   = fcn(xdot_d, l, psid, rd)
xdot = xdot_d - l*sin(psid)*rd;

== matlab function control_clean/track1/yddot_d ==
  data: yddot_d input; l input; psid input; rd input; yddot output; rdot_d input
function yddot   = fcn(yddot_d, l, psid, rd, rdot_d)
yddot = yddot_d + l*cos(psid)*rdot_d - l*sin(psid)*rd*rd;

== matlab function control_clean/track1/ydot ==
  data: u input; v input; r input; psi input; ydot output; l input
function ydot   = fcn(u, v, r, psi, l)
ydot = u*sin(psi)+v*cos(psi)+r*l*cos(psi);

== matlab function control_clean/track1/ydot_d ==
  data: ydot_d input; l input; psid input; rd input; ydot output
function ydot   = fcn(ydot_d, l, psid, rd)
ydot = ydot_d + l*cos(psid)*rd;

== matlab function control_clean/MATLAB Function1 ==
  data: vel input; m parameter; y_v_dot parameter; y_r_dot parameter; n_v_dot parameter; x_u_dot parameter; c_v output
function c_v = coriolis(vel, m, y_v_dot, y_r_dot, n_v_dot,...
x_u_dot)

x = vel(1);
y = vel(2);
z = vel(3);

c_rb = [
    0, 0, -m*y;
    0, 0, m*x;
    m*y, -m*x, 0
];

c_a = [
    0, 0, 2*(y_v_dot*y + z*(y_r_dot + n_v_dot)/2);
    0, 0, -x_u_dot*m*x;
    -2*(y_v_dot*y + z*(y_r_dot + n_v_dot)/2), x_u_dot*m*x, 0
];

c = c_rb + c_a;
c_v = c*vel;

== matlab function control_clean/MATLAB Function ==
  data: eta input; u input; rot_vel output
function rot_vel = rot_mat(eta, u)
theta = eta(3);
J = [cos(theta), -sin(theta), 0;
    sin(theta), cos(theta), 0;
    0, 0, 1];
rot_vel = J*u;

== matlab function control_clean/MATLAB Function2 ==
  data: vel input; d_v output; yvv parameter; yvr parameter; yrv parameter; yrr parameter; nvv parameter; nvr parameter; nrv parameter; nrr parameter; xu output; xuu output; nr output; yv output
function [d_v,xu,xuu,nr,yv] = damping(vel, yvv, yvr, yrv, yrr, nvv, nvr, nrv, nrr)

x = vel(1);
y = vel(2);
z = vel(3);

xu = -25;
xuu = 0;
if(x > 1.2)
    xu = 64.55;
    xuu = -70.92;
end
yv = 0.5*(-40*1000*abs(y))*(1.1+.0045*(1.01/0.09)...
    - 0.1*(0.27/0.09) + 0.016*((0.27/0.09)^2));
yr = 6*(-pi*1000)*sqrt(x^2 + y^2)*0.09^2*1.01;
nv = yr/100;
nr = nv*1.01/3;

d_1 = [
    -xu, 0, 0;
    0, -yv, -yr;
    0, -nv, -nr
];

d_n = [
    xuu*abs(x), 0, 0;
    0, yvv*abs(y) + yvr*abs(z), yrv*abs(y) + yrr*abs(z);
    0, nvv*abs(y) + nvr*abs(z), nrv*abs(y) + nrr*abs(z);
];

d = d_1 - d_n;
d_v = d*vel;

== matlab function control_clean/track2/tracking_ctrl ==
  data: u input; v input; r input; psi input; tu output; fu input; gu input; fv input; fr input; gr input; uax input; uay input; le2x input; le2y input; tr output; l input; xddot_d input; yddot_d input
function [tu,tr]  = fcn(u, v, r, psi, fu, gu, fv, fr, gr, uax, uay, le2x, le2y, l, xddot_d, yddot_d)
gz = [gu*cos(psi), -gr*l*sin(psi); gu*sin(psi), gr*l*cos(psi)];
lep = [le2x; le2y];
f1 = [cos(psi), -sin(psi); sin(psi), cos(psi)];
f2 = [fu - v*r - l*r*r; u*r + fv + l*fr];
fz = f1*f2;
ua = [uax; uay];
ref_ddot = [xddot_d; yddot_d];
uz = inv(gz)*(ref_ddot + lep - fz - ua);
tu = uz(1);
tr = uz(2);

== matlab function control_clean/track2/xddot_d ==
  data: xddot_d input; l input; psid input; rd input; xddot output; rdot_d input
function xddot   = fcn(xddot_d, l, psid, rd, rdot_d)
xddot = xddot_d - l*sin(psid)*rdot_d - l*cos(psid)*rd*rd;
